simulink model "generic_IVS"  (R2024a)
settings: Solver=FixedStepDiscrete  StartTime=0.0  StopTime=inf  FixedStep=0.001  RelTol=1e-3
undefined symbols (not defined in the file): do_waypoints_tail_shifted_2, pathXY, route1_waypoint, route1_waypoint_raw, route2_waypoint, route2_waypoint_raw, route3_waypoint, route3_waypoint_raw, waypoints2
libraries: CarMaker4SL x431, slpidlib x19, dspsigops x3, simulink x1
(part 14 of 15)

== matlab function generic_IVS/CarMaker/Subsystem/Final Project1/Scenario 1/Enabled Subsystem1/MATLAB Function2 ==
  settings: updateMethod=DISCRETE  sampleTime=0.05
  data: waypoints input; startIdx input; global_path_xy_dense output; must1 input; must2 input; goalIdx input
% function global_path_xy_dense = make_global_path(waypoints, startIdx, must1, must2, goalIdx)
% %#codegen
% 
% N = size(waypoints,1);
% max_neighbors = 20;
% MAXLEN = 2000; % 충분히 크게
% 
% % --- via_nodes 처리 ---
% via_nodes = startIdx;
% if must1 ~= 0
%     via_nodes = [via_nodes, must1];
% end
% if must2 ~= 0
%     via_nodes = [via_nodes, must2];
% end
% via_nodes = [via_nodes, goalIdx];
% 
% % --- 진행방향 단위 벡터 계산 ---
% forward_vecs = zeros(N,2);
% for i = 1:N-1
%     v = waypoints(i+1,:) - waypoints(i,:);
%     vn = norm(v);
%     if vn > 1e-6
%         forward_vecs(i,:) = v / vn;
%     else
%         forward_vecs(i,:) = [1,0];
%     end
% end
% forward_vecs(N,:) = forward_vecs(N-1,:);
% 
% % --- 이웃 리스트 (고정 double array) ---
% neighborList = zeros(N, max_neighbors);
% neighborNum  = zeros(N,1);
% D_thresh = 5;
% 
% for i = 1:N
%     dists = sqrt(sum((waypoints - waypoints(i,:)).^2, 2));
%     candidateIdx = find(dists > 0 & dists < D_thresh);
% ncnt = 0;
% for j = 1:length(candidateIdx)
%     idx = candidateIdx(j);
%     vec = waypoints(idx,:) - waypoints(i,:);
%     vn2 = norm(vec);
%     if vn2 < 1e-6
%         continue;
%     end
%     vec = vec / vn2;
%     if dot(forward_vecs(i,:), vec) > 0
%         if ncnt < max_neighbors   % <--- 바꿔주세요!
%             ncnt = ncnt+1;
%             neighborList(i,ncnt) = idx;
%         end
%     end
% end
% neighborNum(i) = ncnt;
% end
% 
% % --- 전체 경로 연결 (via_nodes 순서대로, preallocation) ---
% full_path = zeros(N * (length(via_nodes)-1), 1);
% full_idx = 1;
% 
% for seg = 1:(length(via_nodes)-1)
%     sIdx = via_nodes(seg);
%     gIdx = via_nodes(seg+1);
% 
%     cameFrom = zeros(N,1);
%     gScore   = inf(N,1);
%     fScore   = inf(N,1);
% 
%     gScore(sIdx) = 0;
%     fScore(sIdx) = norm(waypoints(sIdx,:) - waypoints(gIdx,:));
%     openSet = zeros(N,1);
%     openSet(1) = sIdx;
%     openLen = 1;
% 
%     found = false;
%     while openLen > 0
%         fvalues = zeros(openLen,1);
%         for i = 1:openLen
%             fvalues(i) = fScore(openSet(i));
%         end
%         [~, minIdx] = min(fvalues);
%         current = openSet(minIdx);
%         if current == gIdx
%             found = true;
%             break;
%         end
%         if minIdx < openLen
%             openSet(minIdx:openLen-1) = openSet(minIdx+1:openLen);
%         end
%         openLen = openLen - 1;
% 
%         for nidx = 1:neighborNum(current)
%             neighbor = neighborList(current, nidx);
%             edge_cost = norm(waypoints(neighbor,:) - waypoints(current,:));
%             tentative_gScore = gScore(current) + edge_cost;
%             if tentative_gScore < gScore(neighbor)
%                 cameFrom(neighbor) = current;
%                 gScore(neighbor)   = tentative_gScore;
%                 fScore(neighbor)   = tentative_gScore + norm(waypoints(neighbor,:) - waypoints(gIdx,:));
%                 isin = false;
%                 for q = 1:openLen
%                     if openSet(q) == neighbor
%                         isin = true;
%                         break;
%                     end
%                 end
%                 if ~isin && openLen < N
%                     openLen = openLen+1;
%                     openSet(openLen) = neighbor;
%                 end
%             end
%         end
%     end
% 
%     if ~found
%         global_path_xy_dense = zeros(MAXLEN,2); % error 방지
%         return
%     end
% 
%     % --- 경로 추적 (preallocation) ---
%     MAX_PATH_LEN = N;
%     tmp_path = zeros(MAX_PATH_LEN, 1);
%     idx = 1;
%     curr = gIdx;
%     while curr ~= sIdx
%         tmp_path(idx) = curr;
%         curr = cameFrom(curr);
%         idx = idx + 1;
%         if idx > MAX_PATH_LEN
%             break;
%         end
%     end
%     tmp_path(idx) = sIdx;
%     path = tmp_path(idx:-1:1);
% 
%     if seg > 1
%         path = path(2:end);
%     end
% 
%     lenp = length(path);
%     full_path(full_idx : full_idx+lenp-1) = path;
%     full_idx = full_idx + lenp;
% end
% 
% full_path = full_path(1:full_idx-1);
% 
% % --- 경로 좌표 추출 ---
% global_path_xy = waypoints(full_path, :);
% 
% % --- 보간을 통한 촘촘한 경로 생성 ---
% diffs = diff(global_path_xy);
% seg_len = sqrt(sum(diffs.^2, 2));
% s = [0; cumsum(seg_len)];
% ds_interp = 0.5;
% if s(end) < ds_interp
%     interp_xy = global_path_xy;
% else
%     s_interp = (0:ds_interp:s(end))';
%     x_interp = interp1(s, global_path_xy(:,1), s_interp, 'linear');
%     y_interp = interp1(s, global_path_xy(:,2), s_interp, 'linear');
%     interp_xy = [x_interp, y_interp];
% end
% 
% global_path_xy_dense = zeros(MAXLEN,2);
% real_len = size(interp_xy,1);
% if real_len > MAXLEN
%     real_len = MAXLEN;
% end
% global_path_xy_dense(1:real_len,:) = interp_xy(1:real_len,:);
% end


function global_path_xy_dense = make_global_path_with_fsm_sfunc(waypoints, startIdx, must1, must2, goalIdx)
% Simulink에서 사용할 수 있도록 만든 FSM 기반 global path 생성 함수
% 입력:
%   waypoints [Nx2] double, startIdx/must1/must2/goalIdx/state: double scalar
% 출력:
%   global_path_xy_dense [MAXLEN x 2] double

%#codegen

MAXLEN = 2000;
N = size(waypoints,1);

% Simulink 실행 시마다 state=0에서 "한 번만" 새 경로 생성

global_path_xy_dense = gen_global_path(waypoints, startIdx, must1, must2, goalIdx, N, MAXLEN);

end

% ---- 내부 subfunction ----
function global_path_xy_dense = gen_global_path(waypoints, startIdx, must1, must2, goalIdx, N, MAXLEN)

max_neighbors = 20;
% --- via_nodes 처리 ---
via_nodes = startIdx;
if must1 ~= 0
    via_nodes = [via_nodes, must1];
end
if must2 ~= 0
    via_nodes = [via_nodes, must2];
end
via_nodes = [via_nodes, goalIdx];

% --- 진행방향 단위 벡터 계산 ---
forward_vecs = zeros(N,2);
for i = 1:N-1
    v = waypoints(i+1,:) - waypoints(i,:);
    vn = norm(v);
    if vn > 1e-6
        forward_vecs(i,:) = v / vn;
    else
        forward_vecs(i,:) = [1,0];
    end
end
forward_vecs(N,:) = forward_vecs(N-1,:);

% --- 이웃 리스트 ---
neighborList = zeros(N, max_neighbors);
neighborNum  = zeros(N,1);
D_thresh = 5;

for i = 1:N
    dists = sqrt(sum((waypoints - waypoints(i,:)).^2, 2));
    candidateIdx = find(dists > 0 & dists < D_thresh);
    ncnt = 0;
    for j = 1:length(candidateIdx)
        idx = candidateIdx(j);
        vec = waypoints(idx,:) - waypoints(i,:);
        vn2 = norm(vec);
        if vn2 < 1e-6
            continue;
        end
        vec = vec / vn2;
        if dot(forward_vecs(i,:), vec) > 0
            if ncnt < max_neighbors
                ncnt = ncnt+1;
                neighborList(i,ncnt) = idx;
            end
        end
    end
    neighborNum(i) = ncnt;
end

% --- 전체 경로 연결 (via_nodes 순서대로, preallocation) ---
full_path = zeros(N * (length(via_nodes)-1), 1);
full_idx = 1;

for seg = 1:(length(via_nodes)-1)
    sIdx = via_nodes(seg);
    gIdx = via_nodes(seg+1);

    cameFrom = zeros(N,1);
    gScore   = inf(N,1);
    fScore   = inf(N,1);

    gScore(sIdx) = 0;
    fScore(sIdx) = norm(waypoints(sIdx,:) - waypoints(gIdx,:));
    openSet = zeros(N,1);
    openSet(1) = sIdx;
    openLen = 1;

    found = false;
    while openLen > 0
        fvalues = zeros(openLen,1);
        for i = 1:openLen
            fvalues(i) = fScore(openSet(i));
        end
        [~, minIdx] = min(fvalues);
        current = openSet(minIdx);
        if current == gIdx
            found = true;
            break;
        end
        if minIdx < openLen
            openSet(minIdx:openLen-1) = openSet(minIdx+1:openLen);
        end
        openLen = openLen - 1;

        for nidx = 1:neighborNum(current)
            neighbor = neighborList(current, nidx);
            edge_cost = norm(waypoints(neighbor,:) - waypoints(current,:));
            tentative_gScore = gScore(current) + edge_cost;
            if tentative_gScore < gScore(neighbor)
                cameFrom(neighbor) = current;
                gScore(neighbor)   = tentative_gScore;
                fScore(neighbor)   = tentative_gScore + norm(waypoints(neighbor,:) - waypoints(gIdx,:));
                isin = false;
                for q = 1:openLen
                    if openSet(q) == neighbor
                        isin = true;
                        break;
                    end
                end
                if ~isin && openLen < N
                    openLen = openLen+1;
                    openSet(openLen) = neighbor;
                end
            end
        end
    end

    if ~found
        global_path_xy_dense = zeros(MAXLEN,2); % error 방지
        return
    end

    % --- 경로 추적 (preallocation) ---
    MAX_PATH_LEN = N;
    tmp_path = zeros(MAX_PATH_LEN, 1);
    idx = 1;
    curr = gIdx;
    while curr ~= sIdx
        tmp_path(idx) = curr;
        curr = cameFrom(curr);
        idx = idx + 1;
        if idx > MAX_PATH_LEN
            break;
        end
    end
    tmp_path(idx) = sIdx;
    path = tmp_path(idx:-1:1);

    if seg > 1
        path = path(2:end);
    end

    lenp = length(path);
    full_path(full_idx : full_idx+lenp-1) = path;
    full_idx = full_idx + lenp;
end

full_path = full_path(1:full_idx-1);

% --- 경로 좌표 추출 ---
global_path_xy = waypoints(full_path, :);

% --- 보간을 통한 촘촘한 경로 생성 ---
diffs = diff(global_path_xy);
seg_len = sqrt(sum(diffs.^2, 2));
s = [0; cumsum(seg_len)];
ds_interp = 0.5;
if s(end) < ds_interp
    interp_xy = global_path_xy;
else
    s_interp = (0:ds_interp:s(end))';
    x_interp = interp1(s, global_path_xy(:,1), s_interp, 'linear');
    y_interp = interp1(s, global_path_xy(:,2), s_interp, 'linear');
    interp_xy = [x_interp, y_interp];
end

global_path_xy_dense = zeros(MAXLEN,2);
real_len = size(interp_xy,1);
if real_len > MAXLEN
    real_len = MAXLEN;
end
global_path_xy_dense(1:real_len,:) = interp_xy(1:real_len,:);
end

== matlab function generic_IVS/CarMaker/Subsystem/Final Project1/Scenario 1/Enabled Subsystem1/MATLAB Function4 2 ==
  settings: updateMethod=DISCRETE  sampleTime=0.05
  data: waypoints input; local_waypoints_ output; vehicle_position input; head input
function local_waypoints_ = global_to_local_waypoints(waypoints, vehicle_position, head)

    N = size(waypoints, 1);
    local_waypoints_ = zeros(N, 2);

    % 이동 평균 필터 윈도우 크기 설정


    window_size = 18;


    


    % 이동 평균 필터 적용 (x, y 각각)
    x_filtered = movmean(waypoints(:,1), window_size);
    y_filtered = movmean(waypoints(:,2), window_size);

    % 좌표계 변환을 위한 cos/sin
    cos_yaw = cos(-head);
    sin_yaw = sin(-head);

    for i = 1:N
        dx = x_filtered(i) - vehicle_position(1);
        dy = y_filtered(i) - vehicle_position(2);

        local_x = dx * cos_yaw - dy * sin_yaw;
        local_y = dx * sin_yaw + dy * cos_yaw;

        local_waypoints_(i,1) = local_x;
        local_waypoints_(i,2) = local_y;
    end
end

== matlab function generic_IVS/CarMaker/Subsystem/Final Project1/Scenario 1/Enabled Subsystem1/MATLAB Function4 3 ==
  settings: updateMethod=DISCRETE  sampleTime=0.05
  data: global_waypoints input; flag output; x_ego input; y_ego input
function flag  = fsmPathSelectorGlobal( ...
    global_waypoints, ...
    x_ego, y_ego)
%#codegen

% 상태 정의
TRACK_MODE = int32(0);
PARKING_MODE = int32(1);


% 전이 판단용 글로벌 웨이포인트 인덱스 (예: 출발점 근처)
TRIGGER_IDX = 440;  % 예시: global_waypoints(10,:) 기준
DIST_THRESHOLD = 1;  % [m]

% 내부 상태
persistent fsm_state;
if isempty(fsm_state)
    fsm_state = TRACK_MODE;
end

% 트리거 포인트 좌표
trigger_x = global_waypoints(TRIGGER_IDX, 1);
trigger_y = global_waypoints(TRIGGER_IDX, 2);

% 현재 위치와 트리거 지점 사이 거리 계산
dx = trigger_x - x_ego;
dy = trigger_y - y_ego;
dist_to_trigger = sqrt(dx^2 + dy^2);

% FSM 전이 조건
if fsm_state == TRACK_MODE
    if dist_to_trigger < DIST_THRESHOLD
        fsm_state = PARKING_MODE;
    end
end

% 출력 경로 선택
if fsm_state == TRACK_MODE
    flag = 1;
    %goalIdx = 1382;
else
    flag = 0;
    disp('now we are going to parking lot.')
    %goalIdx = 1565;
end

== matlab function generic_IVS/CarMaker/Subsystem/Final Project1/Scenario 1/Enabled Subsystem1/MATLAB Function7 ==
  data: u1 input; target_speed_out output; u2 input; target_speed_in input
% function y = and_logic_latch_permanent(u1, u2)
% %#codegen
% persistent latch;
% if isempty(latch)
%     latch = 0;
% end
% 
% % 정지 조건에 한 번이라도 들어가면 latch=1이 되고, 이후엔 절대 복귀하지 않음
% if (u1 > 5) && (u1 < 6) && (u2 > -38) && (u2 < -35)
%     latch = 1;
% end
% 
% y = latch;
% end



function target_speed_out = and_logic_latch_speed(u1, u2, target_speed_in)
%#codegen
persistent latch;
if isempty(latch)
    latch = 0;
end

% 정지 조건에 한 번이라도 들어가면 latch=1이 되고, 이후엔 절대 복귀하지 않음
if (u1 > 5) && (u1 < 6) && (u2 > -38) && (u2 < -35)
    latch = 1;
end

if latch == 1
    target_speed_out = 0;
else
    target_speed_out = target_speed_in;
end
end

== matlab function generic_IVS/CarMaker/Subsystem/Final Project1/Scenario 1/Enabled Subsystem1/MATLAB Function8 ==
  settings: updateMethod=DISCRETE  sampleTime=0.05
  data: poly_coeff input; lateral_error output; velocity input; lookahead_time input; x_lookahead output; delta_ff output; dy output; d2y output; kappa output
function [lateral_error, x_lookahead, delta_ff, dy, d2y, kappa] = compute_lateral_error_(poly_coeff, velocity, lookahead_time)
% ------------------------------------------------------------
% 경로 다항식 기반 곡률 및 조향각 계산 (스무딩 포함)
% Waypoint 부족 시 조향각 0 처리
% ------------------------------------------------------------

% 휠베이스
L = 3.0;

% Waypoint 부족으로 poly_coeff가 모두 0일 경우 → 계산 중단
if all(poly_coeff == 0)
    lateral_error = 0;
    x_lookahead = velocity * lookahead_time;
    delta_ff = 0;
    dy = 0;
    d2y = 0;
    kappa = 0;
    return;
end

% 다항식 계수 추출
a = 0; b = 0; c = 0; d = 0;
n = length(poly_coeff);
if n == 4
    a = poly_coeff(1); b = poly_coeff(2); c = poly_coeff(3); d = poly_coeff(4);
elseif n == 3
    b = poly_coeff(1); c = poly_coeff(2); d = poly_coeff(3);
elseif n == 2
    c = poly_coeff(1); d = poly_coeff(2);
else
    d = poly_coeff(1);
end

% 1. lateral error (x = 0)
lateral_error = d;

% 2. lookahead 위치
x_lookahead = velocity * lookahead_time;

% 3. dy, d2y
dy = 3*a*x_lookahead^2 + 2*b*x_lookahead + c;
d2y = 6*a*x_lookahead + 2*b;

% 4. kappa 계산 (수치 안정성 보장)
denominator = (1 + dy^2)^(3/2);
if denominator < 1e-6
    denominator = 1e-6;
end
kappa = d2y / denominator;

% 5. 조향각 계산
delta_now = L * kappa;

% 6. Moving Average Filter 적용 (스무딩)
persistent delta_buffer
if isempty(delta_buffer)
    delta_buffer = zeros(1, 30);  % 최근 30개 저장
end

% shift + 최신값 추가
delta_buffer = [delta_now, delta_buffer(1:end-1)];

% 평균값 출력
delta_ff = mean(delta_buffer);

end

== matlab function generic_IVS/CarMaker/Subsystem/Final Project1/Scenario 1/Enabled Subsystem1/MATLAB Function9 ==
  settings: updateMethod=DISCRETE  sampleTime=0.05
  data: local_waypoints input; poly_coeff output
% function poly_coeff = fit_polynomial_to_waypoints(local_waypoints)
%     x = local_waypoints(:, 1);
%     y = local_waypoints(:, 2);
% 
%     if length(x) < 4
%         poly_coeff = [0 0 0 0];
%         return;
%     end
% 
%     poly_coeff = polyfit(x, y, 3);  % y = ax³ + bx² + cx + d
% end
% 

function poly_coeff = fit_polynomial_to_waypoints_(local_waypoints)

% 설정값
poly_order = 3;
max_points = 10;
x_limit = 20;
y_limit = 5;

% 1. x > 0, x < x_limit, |y| < y_limit 필터링
idx = find( ...
    local_waypoints(:,1) > 0 & ...
    local_waypoints(:,1) < x_limit & ...
    abs(local_waypoints(:,2)) < y_limit );

filtered = local_waypoints(idx, :);

% 2. 앞쪽 max_points개만 사용
N = min(max_points, size(filtered, 1));
x = filtered(1:N, 1);
y = filtered(1:N, 2);

% 3. 피팅 수행
if length(x) >= poly_order + 1
    poly_coeff = polyfit(x, y, poly_order);
else
    poly_coeff = zeros(1, 4);
end

end

== matlab function generic_IVS/CarMaker/Subsystem/Final Project1/Scenario 1/Enabled Subsystem1/MATLAB Function12 ==
  data: waypoints input; steering_angle output; vehicle_position input; head input; start_idx output
%% ===== Pure Pursuit 함수 (변경 없음) =====
function [steering_angle, start_idx] = pure_pursuit(waypoints, vehicle_position, head)
    persistent last_target_idx;
    if isempty(last_target_idx), last_target_idx = 1; end

    waypoints_x = waypoints(:,1);
    waypoints_y = waypoints(:,2);


    WHEEL_BASE = 20.0;
    lookahead_dist = 5.5;
    num_points = length(waypoints_x);

    x_ego = vehicle_position(1);
    y_ego = vehicle_position(2);
    local_waypoints = zeros(num_points, 2);

    for i = 1:num_points
        dx = waypoints_x(i) - x_ego;
        dy = waypoints_y(i) - y_ego;
        local_waypoints(i,:) = [ dx*cos(-head)-dy*sin(-head), ...
                                 dx*sin(-head)+dy*cos(-head) ];
    end

    d2 = hypot(waypoints_x - x_ego, waypoints_y - y_ego);
    [~, closest_idx] = min(d2);
    start_idx = max(last_target_idx, closest_idx);

    target_idx = -1;
    for i = start_idx:num_points
        if norm(local_waypoints(i,:))>lookahead_dist && local_waypoints(i,1)>0
            target_idx = i; break;
        end
    end
    if target_idx<0
        for i = 1:start_idx-1
            if norm(local_waypoints(i,:))>lookahead_dist && local_waypoints(i,1)>0
                target_idx = i; break;
            end
        end
    end
    if target_idx<0
        steering_angle = 0; return;
    end

    pt = local_waypoints(target_idx,:);
    alpha = wrapToPi(atan2(pt(2),pt(1)));
    ld = min(max(norm(pt),2.0),20.0);
    steering_angle = atan2(2*WHEEL_BASE*sin(alpha), ld);

    last_target_idx = target_idx;
end

== matlab function generic_IVS/CarMaker/Subsystem/Final Project1/Scenario 1/Enabled Subsystem/MATLAB Function13 ==
  settings: updateMethod=DISCRETE  sampleTime=0.05
  data: gate_flag output boolean size=1; Ego_x input; Ego_y input
function gate_flag = gate_detect(Ego_x, Ego_y)
    % 박스 좌표 설정 (예: 좌상단 기준)
    x_min = -183;  % ← 좌상단 x-183
    x_max = -128;  % ← 우하단 x
    y_min = -164;   % ← 좌하단 y
    y_max = -57;   % ← 좌상단 y -77

    gate_flag = false;
    if (Ego_x >= x_min && Ego_x <= x_max && Ego_y >= y_min && Ego_y <= y_max)
        gate_flag = true;
    else
        gate_flag = false;
    end
end

== matlab function generic_IVS/CarMaker/Subsystem/Final Project1/Scenario 1/Enabled Subsystem/MATLAB Function14 ==
  settings: updateMethod=DISCRETE  sampleTime=0.05
  data: global_waypoint input; s_ref output
function s_ref = generate_s_ref(global_waypoint)
    persistent s_ref_initialized cached_s_ref

    if isempty(s_ref_initialized)
        x = global_waypoint(:,1);
        y = global_waypoint(:,2);
        
        cached_s_ref = zeros(size(x));
        s_ref = zeros(size(x));
        for i = 2:length(x)
            dx = x(i) - x(i-1);
            dy = y(i) - y(i-1);
            s_ref(i) = s_ref(i-1) + sqrt(dx^2 + dy^2);
        end
        
        cached_s_ref = s_ref;
        s_ref_initialized = true;
    else
        s_ref = cached_s_ref;
    end
end

== matlab function generic_IVS/CarMaker/Subsystem/Final Project1/Scenario 1/Enabled Subsystem/MATLAB Function15 ==
  settings: updateMethod=DISCRETE  sampleTime=0.05
  data: ego_pos input; traffic_info input; ego_lane_idx output; wp1 input; wp2 input; wp3 input; traffic_lane_idx output
function [ego_lane_idx, traffic_lane_idx] = get_lane_indices_split(ego_pos, traffic_info, wp1, wp2, wp3)
% ego_pos: [1 x 2]
% traffic_info: [8 x 10] → 각 행: [x, y, vx, vy, ax, ay, yaw, yawRate, length, width]
% wp1~3: [N x 2] (차선별 waypoint 좌표)
% ego_lane_idx: 자차 차선 번호 (1~3)
% traffic_lane_idx: [8 x 1] (각 차량의 차선 번호)

    traffic_pos = traffic_info(:, 1:2);  % x, y 추출
    num_traffic = size(traffic_pos, 1);  % 8 expected
    traffic_lane_idx = zeros(num_traffic, 1);

    % 거리 계산 함수
    function d = min_dist(p, wp)
        dx = wp(:,1) - p(1);
        dy = wp(:,2) - p(2);
        d = min(sqrt(dx.^2 + dy.^2));
    end

    % 자차 차선 판단
    d1 = min_dist(ego_pos, wp1);
    d2 = min_dist(ego_pos, wp2);
    d3 = min_dist(ego_pos, wp3);
    [~, ego_lane_idx] = min([d1, d2, d3]);

    % 트래픽 차량들 차선 판단
    for i = 1:num_traffic
        car_pos = traffic_pos(i, :);
        d1 = min_dist(car_pos, wp1);
        d2 = min_dist(car_pos, wp2);
        d3 = min_dist(car_pos, wp3);
        [~, traffic_lane_idx(i)] = min([d1, d2, d3]);
    end
end

== matlab function generic_IVS/CarMaker/Subsystem/Final Project/Scenario 1/MATLAB Function3 ==
  settings: updateMethod=DISCRETE  sampleTime=1
  data: map_boundary input; mapMatrix output size=[1000, 1000]; traffic_info input; traffic_size input
%% ======== generate_parking_map_ ======== Ver 2025-05-17 10:40
function mapMatrix  = generate_parking_map_(map_boundary, traffic_info, traffic_size)
    %변수설정
    resolution = 1;
    traffic_info_mat = reshape(traffic_info, 5, []).';
    x_values = map_boundary(1:2:end);
    y_values = map_boundary(2:2:end);
    N = size(traffic_info_mat,1);
    w = traffic_size(1);
    h = traffic_size(2);
    x_min = min(x_values);  x_max = max(x_values);
    y_min = min(y_values);  y_max = max(y_values);
    x_size = ceil((x_max-x_min)/resolution);
    y_size = ceil((y_max-y_min)/resolution);
    
    
    mapMatrix = zeros(y_size, x_size); %출력코드
    
    for i = 1:N
        x_c = traffic_info_mat(i, 1);
        y_c = traffic_info_mat(i, 2);
        yaw = traffic_info_mat(i, 3);
        
        dx = w/2;  dy = h/2;
        local = [-dx,-dy; dx,-dy; dx,dy; -dx,dy];
        R = [cos(yaw), -sin(yaw); sin(yaw), cos(yaw)];
        rotated = (R*local')';
        forward_vec = [cos(yaw), sin(yaw)];
        side_vec    = [-sin(yaw), cos(yaw)];
        center = [x_c, y_c] + (w/2)*forward_vec - (h/2)*side_vec;
        corners = rotated + center;
        x_idx = (corners(:,1)-x_min)/resolution + 1;
        y_idx = (y_max-corners(:,2))/resolution + 1;
        mask = poly2mask(x_idx, y_idx, y_size, x_size);
        mapMatrix(mask) = 1;
    end
end

== matlab function generic_IVS/CarMaker/Subsystem/Final Project1/Scenario 1/Enabled Subsystem/MATLAB Function4 1 ==
  settings: updateMethod=DISCRETE  sampleTime=0.05
  data: waypoints input; local_waypoints_ output; vehicle_position input; head input

% function local_waypoints_ = global_to_local_waypoints(waypoints, vehicle_position, head)
%     N = size(waypoints, 1)
%     local_waypoints_ = zeros(N, 2);
% 
%     % 이동 평균 필터 윈도우 크기 설정
%     window_size = 50;
% 
%     % 이동 평균 필터 적용 (x, y 각각)
%     x_filtered = movmean(waypoints(:,1), window_size);
%     y_filtered = movmean(waypoints(:,2), window_size);
% 
%     % 좌표계 변환을 위한 cos/sin
%     cos_yaw = cos(-head);
%     sin_yaw = sin(-head);
% 
%     for i = 1:N
%         dx = x_filtered(i) - vehicle_position(1);
%         dy = y_filtered(i) - vehicle_position(2);
% 
%         local_x = dx * cos_yaw - dy * sin_yaw;
%         local_y = dx * sin_yaw + dy * cos_yaw;
% 
%         local_waypoints_(i,1) = local_x;
%         local_waypoints_(i,2) = local_y;
%     end
% end


% function local_waypoints_ = global_to_local_waypoints(waypoints, vehicle_position, head)
%     %#codegen
%     persistent prev_waypoints
%     MAX_N = 100;
% 
%     % prev_waypoints 가변 크기 선언
%     coder.varsize('prev_waypoints', [MAX_N, 2]);
%     coder.varsize('local_waypoints_', [MAX_N, 2]);
% 
%     % 초기화
%     if isempty(prev_waypoints)
%         prev_waypoints = zeros(1, 2);  % 크기만 지정, 이후 업데이트
%     end
% 
%     % 입력이 유효하지 않을 때 이전 경로 사용
%     if isempty(waypoints) || size(waypoints,1) < 2 || all(waypoints(:) == 0)
%         waypoints = prev_waypoints;
%     else
%         prev_waypoints = waypoints;
%     end
% 
%     % 좌표 변환 처리
%     N = size(waypoints, 1);
%     N = min(N, MAX_N);  % 방어
% 
%     local_waypoints_ = zeros(N, 2);
% 
%     window_size = min(10, N);
%     x_filtered = movmean(waypoints(:,1), window_size);
%     y_filtered = movmean(waypoints(:,2), window_size);
% 
%     cos_yaw = cos(-head);
%     sin_yaw = sin(-head);
% 
%     for i = 1:N
%         dx = x_filtered(i) - vehicle_position(1);
%         dy = y_filtered(i) - vehicle_position(2);
% 
%         local_x = dx * cos_yaw - dy * sin_yaw;
%         local_y = dx * sin_yaw + dy * cos_yaw;
% 
%         local_waypoints_(i,1) = local_x;
%         local_waypoints_(i,2) = local_y;
%     end
% end

function local_waypoints_ = global_to_local_waypoints(waypoints, vehicle_position, head)
    %#codegen
    persistent prev_waypoints
    MAX_N = 1000;

    % 가변 크기 선언
    coder.varsize('prev_waypoints', [MAX_N, 2]);
    coder.varsize('local_waypoints_', [MAX_N, 2]);

    % 초기화
    if isempty(prev_waypoints)
        prev_waypoints = zeros(MAX_N, 2);
    end

    % 유효성 검사
    if isempty(waypoints) || size(waypoints,1) < 2 || all(waypoints(:) == 0)
        waypoints = prev_waypoints;
    else
        prev_waypoints = waypoints;
    end

    % 길이 확인
    N = size(waypoints, 1);
    N = min(N, MAX_N);

    local_waypoints_ = zeros(N, 2);

    % 🔧 이동 평균 필터 OFF
    x_data = waypoints(:,1);
    y_data = waypoints(:,2);

    % 좌표 변환
    cos_yaw = cos(-head);
    sin_yaw = sin(-head);

    for i = 1:N
        dx = x_data(i) - vehicle_position(1);
        dy = y_data(i) - vehicle_position(2);

        local_x = dx * cos_yaw - dy * sin_yaw;
        local_y = dx * sin_yaw + dy * cos_yaw;

        local_waypoints_(i,1) = local_x;
        local_waypoints_(i,2) = local_y;
    end
end

== matlab function generic_IVS/CarMaker/Subsystem/Final Project1/Scenario 1/Enabled Subsystem/MATLAB Function6 ==
  settings: updateMethod=DISCRETE  sampleTime=0.05
  data: s_ref input; global_path output; global_waypoint_2 input; Ego_x input; Ego_y input; Ego_Yaw input; Ego_Vx input; Ego_Ax input; target_speed input; obs_pre input; TargetTolgateLane input; gate_flag input
function global_path  = trajectory_path(s_ref, global_waypoint_2, Ego_x, Ego_y, Ego_Yaw, Ego_Vx, Ego_Ax, target_speed, obs_pre, TargetTolgateLane, gate_flag)
    LANE_WIDTH = 3.0;
    CENTER_LANE = 2;
    TargetTolgateLane_d = (TargetTolgateLane - CENTER_LANE) * LANE_WIDTH;



    mapx= global_waypoint_2(:,1);
    mapy= global_waypoint_2(:,2);
    
    % === 초기 자차 위치 및 상태 === %
    
    obs=obs_pre(:,[1:2]);

    x0 = Ego_x; %
    y0 = Ego_y; %
    yaw0 = Ego_Yaw; % 
    v0 = Ego_Vx; a0 = Ego_Ax; %% 초기값 

    % 1. Frenet 좌표계 위치 (s0, d0) 계산
    [s0, d0] = get_frenet(x0, y0, mapx, mapy);

    % 2. 기준 경로에서의 진행 방향 (yaw_path) 계산
    [~, ~, yaw_path] = get_cartesian(s0, d0, mapx, mapy, s_ref);

    % 3. 경로 기준 상대 진행 방향 계산
    yawi = yaw0 - yaw_path;

    % 4. Frenet 상태 초기값
    si    = s0;
    si_d  = v0 * cos(yawi);
    si_dd = a0 * cos(yawi);
    sf_d  = target_speed; %%%%%%%%%%%%%%%%%%%%%%%%%%%%%%%%%%%%%%%%%%%
    sf_dd = 0;

    di    = d0;
    di_d  = v0 * sin(yawi);
    di_dd = a0 * sin(yawi);
    df_d  = 0;
    df_dd = 0;

    opt_d = di;  % 횡 방향 목표 유지
    
    %% 
   
    [path, opt_ind] = frenet_optimal_planning(...
                                              si, si_d, si_dd, sf_d, sf_dd, di, di_d, di_dd, ...
                                              df_d, df_dd, obs, mapx, mapy, s_ref, opt_d, gate_flag, TargetTolgateLane_d); %%%%%%%%%%%%%%%%%%%%%%%%%%%%%%%%obs 만처리하면됨 
   
    %% 출력
    global_path = [path(opt_ind).x(1:path(opt_ind).len)', path(opt_ind).y(1:path(opt_ind).len)'];  % N×2
    
    

    % % === 디버깅용 시각화 ===
    % figure(1); clf; hold on; axis equal;
    % plot(mapx, mapy, 'k--'); % 기준 경로
    % plot(global_path(:,1), global_path(:,2), 'b-', 'LineWidth', 2); % 최적 궤적
    % plot(Ego_x, Ego_y, 'ro'); % 자차 현재 위치
    % title('Selected Optimal Trajectory');
    % grid on;

    
end

function [path, opt_ind] = frenet_optimal_planning(...
                                                  si, si_d, si_dd, sf_d, sf_dd, di, di_d, di_dd, ...
                                                  df_d, df_dd, obs, mapx, mapy, s_ref, opt_d, gate_flag, TargetTolgateLane_d)
    % 1. Frenet 궤적 후보 생성
    [fplist, MAX_len, LENG_path] = calc_frenet_paths(...
                                                    si, si_d, si_dd, sf_d, sf_dd, di, di_d, di_dd, ...
                                                    df_d, df_dd, opt_d, gate_flag, TargetTolgateLane_d);


    % 2. Global 궤적 변환
    fplist = calc_global_paths(fplist, mapx, mapy, s_ref);

    % 3. 제약조건 및 충돌 검사 → 유효 trajectory만 반환
    [valid_paths, num_valid] = check_path(fplist, obs, MAX_len, LENG_path);

    % 4. 최적 경로 선택
    min_cost = inf;
    opt_ind = 1;  % 초기값

    for i = 1:num_valid
        if valid_paths(i).c_tot < min_cost
            min_cost = valid_paths(i).c_tot;
            opt_ind = i;
        end
    end

    % 5. 출력 (최종 유효 경로들)
    path = valid_paths;
end

    

function [fplist, MAX_len, LENG_path] = calc_frenet_paths(...
                                                            si, si_d, si_dd, sf_d, sf_dd, di, di_d, di_dd, ...
                                                            df_d, df_dd, opt_d, gate_flag, TargetTolgateLane_d)
  
    % % 차선 번호(1,2,3)를 실제 Frenet d 좌표로 변환
    % LANE_WIDTH = 3;     % 실제 차선 폭 [m]
    % CENTER_LANE = 2;      % 중앙 차선 번호
    % TargetTolgateLane_d = (TargetTolgateLane - CENTER_LANE) * LANE_WIDTH;


    
    TARGET_SPEED = sf_d;
    DF_SET = linspace(-3, 3, 3); 
    DT = 0.05; 
    DT_T = 0.2; 
    MIN_T = 2; 
    MAX_T = 4; 
     % K_J Jerk 웨이트 s,d 둘다 , K_T t_f에 대한 항, K_D Diff d에대한 diff, K_V s에 대한 diff(속도 s_d에 대한 diff)
    MAX_len= (MAX_T/DT)+1;

    K_J = 0.1; K_T = 1; K_D = 1; K_V = 1;

    W_LAT = 1.0; W_LON = 1.0; %종방향 횡방향 웨이트
    
    LENG_path = 3*(MAX_T-MIN_T)/DT_T; 
    fp_templet = struct( ...
    't', zeros(1,MAX_len), ...
    'd', zeros(1,MAX_len), 'd_d', zeros(1,MAX_len), 'd_dd', zeros(1,MAX_len), 'd_ddd', zeros(1,MAX_len), ...
    's', zeros(1,MAX_len), 's_d', zeros(1,MAX_len), 's_dd', zeros(1,MAX_len), 's_ddd', zeros(1,MAX_len), ...
    'c_lat', 0, 'c_lon', 0, 'c_tot', 0, ...
    'x', zeros(1,MAX_len), 'y', zeros(1,MAX_len), 'yaw', zeros(1,MAX_len), ...
    'ds', zeros(1,MAX_len), 'kappa', zeros(1,MAX_len), ...
    'len', 0);

    fplist = repmat(fp_templet, 1, LENG_path);  % 빈 구조체 배열로 초기화
    index=1;
    for df = DF_SET
        for T = MIN_T:DT_T:MAX_T
            
            % Lateral trajectory (Quintic)
            [a0_d, a1_d, a2_d, a3_d, a4_d, a5_d] = calc_quintic(di, di_d, di_dd, df, df_d, df_dd, T);
            
            t = 0:DT:T;
            
            d = a0_d + a1_d*t + a2_d*t.^2 + a3_d*t.^3 + a4_d*t.^4 + a5_d*t.^5;
            d_d = a1_d + 2*a2_d*t + 3*a3_d*t.^2 + 4*a4_d*t.^3 + 5*a5_d*t.^4;
            d_dd = 2*a2_d + 6*a3_d*t + 12*a4_d*t.^2 + 20*a5_d*t.^3;
            d_ddd = 6*a3_d + 24*a4_d*t + 60*a5_d*t.^2;
            
            
            % Longitudinal trajectory (Quartic)
            %sf_d에 Target Speed를 기준으로 여러개 생성해야된다
            %sf 인자는 어디로 갔나
            [a0_s, a1_s, a2_s, a3_s, a4_s] = calc_quartic(si, si_d, si_dd, sf_d, sf_dd, T);
            s = a0_s + a1_s*t + a2_s*t.^2 + a3_s*t.^3 + a4_s*t.^4;
            s_d = a1_s + 2*a2_s*t + 3*a3_s*t.^2 + 4*a4_s*t.^3;
            s_dd = 2*a2_s + 6*a3_s*t + 12*a4_s*t.^2;
            s_ddd = 6*a3_s + 24*a4_s*t;
            
           
            %% 비용 계산
            J_lat = sum(d_ddd.^2); %적분항 인데 왜 T로 안나눠 임마 
            J_lon = sum(s_ddd.^2); %적분항 
            if gate_flag
                d_gate_weight = 10000000000;
                d_diff = (d(end) - TargetTolgateLane_d)^2 * d_gate_weight;
            else
                d_diff = (d(end) - opt_d)^2;
            end

            % if gate_flag
            %     opt_d = TargetTolgateLane_d;
            % else
            %     opt_d = di;
            % end


            s_diff = (TARGET_SPEED - s_d(end))^2; %ACC랑 최대한 유지하기 위함

            
            % if gate_flag
            %     d_gate_weight = 10000000000;
            %     d_diff = (d(end) - TargetTolgateLane_d)^2 * d_gate_weight;
            %     fprintf('[DEBUG] df = %.2f | d(end) = %.2f | target_d = %.2f | cost = %.2e\n', ...
            %             df, d(end), TargetTolgateLane_d, d_diff);
            % else
            %     d_diff = (d(end) - opt_d)^2;
            % end

            %% 비용함수
            c_lat = K_J * J_lat  + K_D * d_diff + K_T * T; %% cost_lateral
            c_lon = K_J * J_lon  + K_V * s_diff + K_T * T; %% cost_longitual
            c_tot = W_LAT * c_lat + W_LON * c_lon; %% total Cost가 낮은것을 선택

            len = length(t);  % ← 이 줄이 꼭 필요!

            % 1. fp 템플릿 기반 새 구조체 생성
            fp = fp_templet;

            % 2. 유효 길이 저장
            fp.len = len;

            % 3. 시간 및 궤적 데이터 복사
            fp.t(1:len)     = t;
            fp.d(1:len)     = d;
            fp.d_d(1:len)   = d_d;
            fp.d_dd(1:len)  = d_dd;
            fp.d_ddd(1:len) = d_ddd;

            fp.s(1:len)     = s;
            fp.s_d(1:len)   = s_d;
            fp.s_dd(1:len)  = s_dd;
            fp.s_ddd(1:len) = s_ddd;

            % 4. 비용도 할당
            fp.c_lat = c_lat;
            fp.c_lon = c_lon;
            fp.c_tot = c_tot;

            % 5. fplist에 대입
            fplist(index) = fp;
            if(index<LENG_path)
            index = index +1;
            end
        end
    end
end

function fplist = calc_global_paths(fplist, mapx, mapy, s_ref)
    for i = 1:length(fplist)
        fp = fplist(i);
        len = fp.len;

        % === Global 좌표 변환 === %
        for j = 1:len
            [fp.x(j), fp.y(j), ~] = get_cartesian(fp.s(j), fp.d(j), mapx, mapy, s_ref);
        end

        % === Yaw, ds 계산 === %
        for j = 1:len-1
            dx = fp.x(j+1) - fp.x(j);
            dy = fp.y(j+1) - fp.y(j);
            fp.yaw(j) = atan2(dy, dx);
            fp.ds(j) = hypot(dx, dy);
        end
        if len >= 2
            fp.yaw(len) = fp.yaw(len - 1);
            fp.ds(len)  = fp.ds(len - 1);
        else
            fp.yaw(len) = 0;
            fp.ds(len)  = 1e-6;  % 너무 작지 않게 보호
        end

        % === 곡률 계산 === %
        for j = 1:len-1
            dyaw = atan2(sin(fp.yaw(j+1) - fp.yaw(j)), cos(fp.yaw(j+1) - fp.yaw(j)));
            fp.kappa(j) = dyaw / fp.ds(j);
        end
        if len >= 2
            fp.kappa(len) = fp.kappa(len - 1);
        else
            fp.kappa(len) = 0;
        end

        % 업데이트된 fp 구조체 다시 저장
        fplist(i) = fp;
    end
end

function [valid_paths, numValid] = check_path(fplist, obs, MAX_len, LENG_path)
    % 정적 템플릿 구조체 선언
    fp_templet = struct( ...
        't', zeros(1,MAX_len), ...
        'd', zeros(1,MAX_len), 'd_d', zeros(1,MAX_len), 'd_dd', zeros(1,MAX_len), 'd_ddd', zeros(1,MAX_len), ...
        's', zeros(1,MAX_len), 's_d', zeros(1,MAX_len), 's_dd', zeros(1,MAX_len), 's_ddd', zeros(1,MAX_len), ...
        'c_lat', 0, 'c_lon', 0, 'c_tot', 0, ...
        'x', zeros(1,MAX_len), 'y', zeros(1,MAX_len), 'yaw', zeros(1,MAX_len), ...
        'ds', zeros(1,MAX_len), 'kappa', zeros(1,MAX_len), ...
        'len', 0);

    % 제약 조건
    V_MAX = 30;
    ACC_MAX = 5;
    K_MAX = 1.5;

    % 고정 크기 구조체 배열 선언
    valid_paths = repmat(fp_templet, 1, LENG_path);
    index = 1;
    numValid = 0;

    for i = 1:length(fplist)
        fp = fplist(i);
        len = fp.len;

        acc_squared = fp.s_dd(1:len).^2;  % s 방향에 대한 가속도만 고려
        

        if all(fp.s_d(1:len) > V_MAX)

            continue;
        elseif any(acc_squared > ACC_MAX^2)
            continue;
        elseif any(abs(fp.kappa(1:len)) > K_MAX)
            continue;
        elseif collision_check(fp, obs)
            continue;
        elseif any(abs(fp.d(1:len)) > 3.8)
            continue;
        else
            valid_paths(index) = fp;
            index = index + 1;
            numValid = numValid + 1;
        end
    end

end


function collision = collision_check(fp, obs_global)
    CAR_RADIUS = 2;
    OBSTACLE_RADIUS = 1;% rad default 0.5
    SAFE_DIST_SQ = (CAR_RADIUS + OBSTACLE_RADIUS)^2;

    len = fp.len;
    collision = false;

    for i = 1:size(obs_global, 1)
        dx = fp.x(1:len) - obs_global(i,1);
        dy = fp.y(1:len) - obs_global(i,2);
        dists_sq = dx.^2 + dy.^2;

        if any(dists_sq <= SAFE_DIST_SQ)
            collision = true;
            return;
        end
    end
end



function [s, d] = get_frenet(x, y, x_ref, y_ref)
    idx = get_closest_waypoint(x, y, x_ref, y_ref);
    if idx == 1
        prev_idx = 1; next_idx = 2;
    elseif idx == length(x_ref)
        prev_idx = length(x_ref) - 1; next_idx = length(x_ref);
    else
        prev_idx = idx - 1; next_idx = idx;
    end
    vec_path = [x_ref(next_idx) - x_ref(prev_idx); y_ref(next_idx) - y_ref(prev_idx)];
    vec_ego  = [x - x_ref(prev_idx); y - y_ref(prev_idx)];
    proj = dot(vec_path, vec_ego) / norm(vec_path)^2 * vec_path;
    perp = vec_ego - proj;
    d = norm(perp);
    if det([vec_path, vec_ego]) < 0
        d = -d;
    end
    s = 0;
    for i = 1:(prev_idx - 1)
        s = s + norm([x_ref(i+1) - x_ref(i), y_ref(i+1) - y_ref(i)]);
    end
    s = s + norm(proj);
end

function [x, y, heading] = get_cartesian(s, d, x_ref, y_ref, s_ref)
    s = mod(s, s_ref(end));
    idx = find(s_ref <= s, 1, 'last');
    if idx >= length(s_ref), idx = length(s_ref) - 1; end
    dx = x_ref(idx+1) - x_ref(idx);
    dy = y_ref(idx+1) - y_ref(idx);
    heading = atan2(dy, dx);
    ds = s - s_ref(idx);
    x_base = x_ref(idx) + ds * cos(heading);
    y_base = y_ref(idx) + ds * sin(heading);
    x = x_base + d * cos(heading + pi/2);
    y = y_base + d * sin(heading + pi/2);
end

function idx = get_closest_waypoint(x, y, x_ref, y_ref)
    dists = sqrt((x_ref - x).^2 + (y_ref - y).^2);
    [~, idx] = min(dists);
end

function [a0, a1, a2, a3, a4, a5] = calc_quintic(xi, vi, ai, xf, vf, af, T)
    a0 = xi;
    a1 = vi;
    a2 = 0.5 * ai;
    A = [T^3, T^4, T^5;
         3*T^2, 4*T^3, 5*T^4;
         6*T, 12*T^2, 20*T^3];
    b = [xf - a0 - a1*T - a2*T^2;
         vf - a1 - 2*a2*T;
         af - 2*a2];
    x = A\b;
    a3 = x(1); a4 = x(2); a5 = x(3);
end

function [a0, a1, a2, a3, a4] = calc_quartic(xi, vi, ai, vf, af, T)
    a0 = xi;
    a1 = vi;
    a2 = 0.5 * ai;
    A = [3*T^2, 4*T^3;
         6*T, 12*T^2];
    b = [vf - a1 - 2*a2*T;
         af - 2*a2];
    x = A\b;
    a3 = x(1); a4 = x(2);
end

== matlab function generic_IVS/CarMaker/Subsystem/Final Project1/Scenario 1/Enabled Subsystem/MATLAB Function8 ==
  settings: updateMethod=DISCRETE  sampleTime=0.05
  data: poly_coeff input; lateral_error output; velocity input; lookahead_time input; x_lookahead output; delta_ff output; dy output; d2y output; kappa output
% function [lateral_error, x_lookahead, delta_ff, dy, d2y, kappa] = compute_lateral_error_(poly_coeff, velocity, lookahead_time)
% % ------------------------------------------------------------
% % 경로 다항식 기반 곡률 및 조향각 계산 (스무딩 포함)
% % Waypoint 부족 시 조향각 0 처리
% % ------------------------------------------------------------
% 
% % 휠베이스
% L = 2.9;
% 
% % Waypoint 부족으로 poly_coeff가 모두 0일 경우 → 계산 중단
% if all(poly_coeff == 0)
%     lateral_error = 0;
%     x_lookahead = velocity * lookahead_time;
%     delta_ff = 0;
%     dy = 0;
%     d2y = 0;
%     kappa = 0;
%     return;
% end
% 
% % 다항식 계수 추출
% a = 0; b = 0; c = 0; d = 0;
% n = length(poly_coeff);
% if n == 4
%     a = poly_coeff(1); b = poly_coeff(2); c = poly_coeff(3); d = poly_coeff(4);
% elseif n == 3
%     b = poly_coeff(1); c = poly_coeff(2); d = poly_coeff(3);
% elseif n == 2
%     c = poly_coeff(1); d = poly_coeff(2);
% else
%     d = poly_coeff(1);
% end
% 
% % 1. lateral error (x = 0)
% lateral_error = d;
% 
% % 2. lookahead 위치
% x_lookahead = velocity * lookahead_time;
% 
% % 3. dy, d2y
% dy = 3*a*x_lookahead^2 + 2*b*x_lookahead + c;
% d2y = 6*a*x_lookahead + 2*b;
% 
% % 4. kappa 계산 (수치 안정성 보장)
% denominator = (1 + dy^2)^(3/2);
% if denominator < 1e-6
%     denominator = 1e-6;
% end
% kappa = d2y / denominator;
% 
% % 5. 조향각 계산
% delta_now = L * kappa;
% 
% % 6. Moving Average Filter 적용 (스무딩)
% persistent delta_buffer
% if isempty(delta_buffer)
%     delta_buffer = zeros(1, 30);  % 최근 30개 저장
% end
% 
% % shift + 최신값 추가
% delta_buffer = [delta_now, delta_buffer(1:end-1)];
% 
% % 평균값 출력
% delta_ff = mean(delta_buffer);
% 
% end
function [lateral_error, x_lookahead, delta_ff, dy, d2y, kappa] = compute_lateral_error_(poly_coeff, velocity, lookahead_time)
% ------------------------------------------------------------
% 경로 다항식 기반 곡률 및 조향각 계산 (필터 제거 버전)
% ------------------------------------------------------------

% 휠베이스
L = 2.9;

% 웨이포인트가 없으면 무효 처리
if all(poly_coeff == 0)
    lateral_error = 0;
    x_lookahead = velocity * lookahead_time;
    delta_ff = 0;
    dy = 0;
    d2y = 0;
    kappa = 0;
    return;
end

% 다항식 계수 추출
a = 0; b = 0; c = 0; d = 0;
n = length(poly_coeff);
if n == 4
    a = poly_coeff(1); b = poly_coeff(2); c = poly_coeff(3); d = poly_coeff(4);
elseif n == 3
    b = poly_coeff(1); c = poly_coeff(2); d = poly_coeff(3);
elseif n == 2
    c = poly_coeff(1); d = poly_coeff(2);
else
    d = poly_coeff(1);
end

% 1. lateral error (x = 0 기준)
lateral_error = d;

% 2. lookahead 위치
x_lookahead = velocity * lookahead_time;

% 3. 경사도 및 곡률 미분값 계산
dy = 3*a*x_lookahead^2 + 2*b*x_lookahead + c;
d2y = 6*a*x_lookahead + 2*b;

% 4. 곡률 계산
denominator = (1 + dy^2)^(3/2);
if denominator < 1e-6
    denominator = 1e-6;
end
kappa = d2y / denominator;

% 5. 조향각 = 휠베이스 × 곡률
delta_now = L * kappa;

% 6. 필터 제거 → 바로 적용
delta_ff = delta_now;

end

== matlab function generic_IVS/CarMaker/Subsystem/Final Project1/Scenario 1/Enabled Subsystem2/MATLAB Function11 ==
  settings: updateMethod=DISCRETE  sampleTime=0.05
  data: obstacle_info input; start_point input; goal_point input; x_path output; y_path output
function [x_path, y_path] = rrt_path_planner(obstacle_info, start_point, goal_point)
%#codegen
    persistent success_cached x_path_cached y_path_cached
    MAX_PATH_LEN = 500;
    
    %--- 캐시 초기화 및 반환 로직 ---
    if isempty(success_cached)
        % 처음 호출될 때
        success_cached  = false;
        x_path_cached   = zeros(MAX_PATH_LEN,1);
        y_path_cached   = zeros(MAX_PATH_LEN,1);
    elseif success_cached
        % 이미 성공적으로 계산된 경로가 있으면 바로 반환
        x_path = x_path_cached;
        y_path = y_path_cached;
        return;
    end

    %%RRT*
    MAX_NODES    = 2000;
    goal_radius  = 3.0;
    goal_sample_rate = 0.15;
    eta          = 2.0;

    start = [start_point(1), start_point(2)];
    finish_point  = [goal_point(1),  goal_point(2)];
    vehicle_h_w = [1.47, 3.1];
    %vehicle_h_w = [2.1, 4.6];
    map_boundary = [5.5, -4, 47.5, -3.9, 47.5, -44.9, 5.5, -44.9];
    x_vals = map_boundary(1:2:end);
    y_vals = map_boundary(2:2:end);
    x_min = min(x_vals); x_max = max(x_vals);
    y_min = min(y_vals); y_max = max(y_vals);

    % 장애물 정보 파싱 (5개씩)
    if mod(length(obstacle_info),5) ~= 0
        obstacles = zeros(0,5);
    else
        num_obj = int32(floor(length(obstacle_info)/5));
        data = reshape(obstacle_info,[5, num_obj])';
        obstacles = [data(:,1), data(:,2), data(:,5), data(:,4), data(:,3)];
    end

    empty_node = struct('pos',zeros(1,2),'cost',0,'parent',int32(0));
    nodes = repmat(empty_node, MAX_NODES, 1);
    nodes(1).pos = start;
    node_count = int32(1);
    goal_node  = int32(0);

    % 샘플링 반복
    for iter = 1:2000
        if rand < goal_sample_rate
            sample = finish_point;
        else
            sample = [x_min + rand*(x_max-x_min), y_min + rand*(y_max-y_min)];
        end
        % 최근접 노드 찾기
        nearest_idx = int32(1);
        min_dist = norm(nodes(1).pos - sample);
        for i = 2:node_count
            d = norm(nodes(i).pos - sample);
            if d < min_dist
                min_dist = d;
                nearest_idx = int32(i);
            end
        end
        % 새 노드 생성
        dir_vec = sample - nodes(nearest_idx).pos;
        dist = norm(dir_vec);
        if dist > eta
            dir_vec = dir_vec / dist * eta;
        end
        new_pos = nodes(nearest_idx).pos + dir_vec;
        % 충돌 체크
        if check_collision(nodes(nearest_idx).pos, new_pos, vehicle_h_w, obstacles)
            continue;
        end
        % 노드 추가
        node_count = node_count + 1;
        if node_count > MAX_NODES, break; end
        nodes(node_count).pos    = new_pos;
        nodes(node_count).cost   = nodes(nearest_idx).cost + dist;
        nodes(node_count).parent = nearest_idx;
        % 목표 반경 체크
        if norm(new_pos - finish_point) < goal_radius
            goal_node = node_count;
            break;
        end
    end

    if goal_node > 0
        idx = goal_node; i = 0;
        temp_path = zeros(MAX_PATH_LEN,2);
        while idx>0 && i<MAX_PATH_LEN
            i = i + 1;
            temp_path(i,:) = nodes(idx).pos;
            idx = nodes(idx).parent;
        end
        flipped = flipud(temp_path(1:i,:));
        pre_steps  = 10; post_steps = 8; step_dist = 0.5;
        last_pos = flipped(end,:);
        if last_pos(1) < finish_point(1)
            hybrid_x = finish_point(1) - 0.9;
        else
            hybrid_x = finish_point(1) + 0.9;
        end
        if finish_point(2) > -36.5
            pre_path  = [ repmat(hybrid_x,pre_steps,1), finish_point(2)-step_dist*(pre_steps:-1:1)'];
            post_path = [ repmat(hybrid_x,post_steps,1), finish_point(2)+step_dist*(1:post_steps)' ];
        else
            pre_path  = [ repmat(hybrid_x,pre_steps,1), finish_point(2)+step_dist*(pre_steps:-1:1)'];
            post_path = [ repmat(hybrid_x,post_steps,1), finish_point(2)-step_dist*(1:post_steps)' ];
        end
        hybrid_path = [pre_path; finish_point; post_path];

        raw_path   = [flipped; hybrid_path];
        path_interp = smooth_path(raw_path, 0.5);
        path_interp = smooth_moving_average(path_interp, 20);

        % 최종 경로
        path_len = size(path_interp,1);
        path_out = zeros(MAX_PATH_LEN,2);
        path_out(1:path_len,:) = path_interp;

        % x,y 분리 및 캐싱
        x_path = path_out(:,1);
        y_path = path_out(:,2);
        x_path_cached  = x_path;
        y_path_cached  = y_path;
        success_cached = true;
    else
        % 실패 시 빈 벡터
        x_path = zeros(MAX_PATH_LEN,1);
        y_path = zeros(MAX_PATH_LEN,1);
    end
end

%% ===== 보조 함수
function collision = check_collision(p1, p2, vehicle_size, obs_list)
    collision = false;
    steps = 10;
    exception_obs = [26.5, -4, 0.1, 42.0, 0];
    for t = linspace(0,1,steps)
        pt = (1-t)*p1 + t*p2;
        yaw = atan2(p2(2)-p1(2), p2(1)-p1(1));
        veh = get_bbox(pt, yaw, vehicle_size);
        for i = 1:size(obs_list,1)
            if check_single_collision(veh, obs_list(i,:))
                collision = true; return;
            end
        end
        if check_single_collision(veh, exception_obs)
            collision = true; return;
        end
    end
end

function smoothed = smooth_moving_average(path, windowSize)
    N = size(path,1);
    half = floor(windowSize/2);
    smoothed = zeros(N,2);

    for i = 1:N
        if i == 1 || i == N
            smoothed(i,:) = path(i,:);  % 시작점과 끝점은 고정
        else
            i0 = max(1, i-half);
            i1 = min(N, i+half);
            smoothed(i,:) = mean(path(i0:i1,:), 1);
        end
    end
end

function is_collide = check_single_collision(veh_box, obs)
    yaw_obs = obs(5);
    rear_center = obs(1:2);
    length_obs = obs(4);
    width_obs = obs(3);
    fwd_vec = [cos(yaw_obs), sin(yaw_obs)];
    center = rear_center + (length_obs/2) * fwd_vec;
    obs_box = get_bbox(center, yaw_obs, [width_obs, length_obs]);
    is_collide = box_overlap(veh_box, obs_box);
end

function box = get_bbox(center, yaw, size)
    w = size(1); h = size(2);
    dx = [ w/2, -w/2, -w/2,  w/2];
    dy = [ h/2,  h/2, -h/2, -h/2];
    R = [cos(yaw), -sin(yaw); sin(yaw), cos(yaw)];
    temp = R * [dx; dy];
    box = temp + center';
end

function overlap = box_overlap(b1, b2)
    overlap = true;
    axes = get_axes(b1, b2);
    for i = 1:size(axes,2)
        proj1 = axes(:,i)' * b1;
        proj2 = axes(:,i)' * b2;
        if max(proj1) < min(proj2) || max(proj2) < min(proj1)
            overlap = false;
            return;
        end
    end
end

function axes = get_axes(b1, b2)
    edges = [b1(:,2)-b1(:,1), b1(:,3)-b1(:,2)];
    normals = [-edges(2,:); edges(1,:)];
    axes = normals ./ vecnorm(normals);
end

function path_smooth = smooth_path(path_raw, step_size)
    if size(path_raw, 1) < 2
        path_smooth = path_raw;
        return;
    end
    dist = [0; cumsum(vecnorm(diff(path_raw), 2, 2))];
    query = 0:step_size:dist(end);
    if query(end) < dist(end)
        query(end+1) = dist(end);
    end
    x_interp = spline(dist, path_raw(:,1), query);
    y_interp = spline(dist, path_raw(:,2), query);
    path_smooth = [x_interp', y_interp'];
end
